simulink model "TorqueVectoringAllocatorTestWrapper"  (R2026b)
settings: Solver=FixedStepDiscrete  StopTime=1.0  FixedStep=TorqueVectoringControlSampleTime
settings Model: DataDictionary=VehicleData.sldd  Creator=Xu Dingyi  LastModifiedBy=29358
settings DebuggingCC: AlgebraicLoopMsg=error

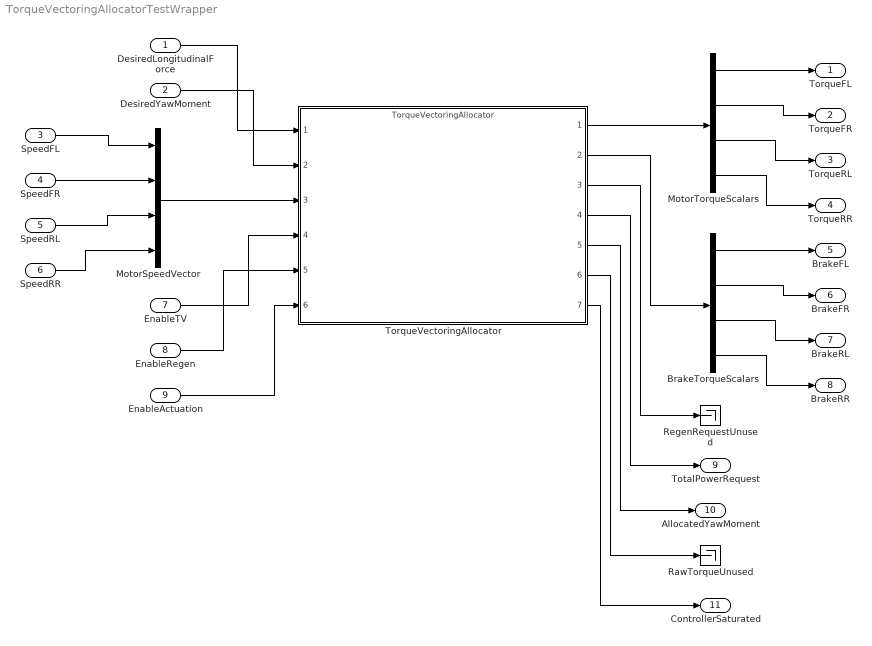
== system TorqueVectoringAllocatorTestWrapper ==
  DesiredLongitudinalForce : Inport  OutDataTypeStr=double  Unit=N
  DesiredYawMoment : Inport  Port=2  OutDataTypeStr=double  Unit=N*m
  SpeedFL : Inport  Port=3  OutDataTypeStr=double  Unit=rad/s
  SpeedFR : Inport  Port=4  OutDataTypeStr=double  Unit=rad/s
  SpeedRL : Inport  Port=5  OutDataTypeStr=double  Unit=rad/s
  SpeedRR : Inport  Port=6  OutDataTypeStr=double  Unit=rad/s
  EnableTV : Inport  Port=7  OutDataTypeStr=boolean
  EnableRegen : Inport  Port=8  OutDataTypeStr=boolean
  EnableActuation : Inport  Port=9  OutDataTypeStr=boolean
  BrakeTorqueScalars : Demux
  MotorSpeedVector : Mux
  MotorTorqueScalars : Demux
  RawTorqueUnused : Terminator
  RegenRequestUnused : Terminator
  TorqueVectoringAllocator : ModelReference  ModelNameDialog=TorqueVectoringAllocator  ModelReferenceVersion=2.0
  TorqueFL : Outport  OutDataTypeStr=double  Unit=N*m
  TorqueFR : Outport  Port=2  OutDataTypeStr=double  Unit=N*m
  TorqueRL : Outport  Port=3  OutDataTypeStr=double  Unit=N*m
  TorqueRR : Outport  Port=4  OutDataTypeStr=double  Unit=N*m
  BrakeFL : Outport  Port=5  OutDataTypeStr=double  Unit=N*m
  BrakeFR : Outport  Port=6  OutDataTypeStr=double  Unit=N*m
  BrakeRL : Outport  Port=7  OutDataTypeStr=double  Unit=N*m
  BrakeRR : Outport  Port=8  OutDataTypeStr=double  Unit=N*m
  TotalPowerRequest : Outport  Port=9  OutDataTypeStr=double  Unit=W
  AllocatedYawMoment : Outport  Port=10  OutDataTypeStr=double  Unit=N*m
  ControllerSaturated : Outport  Port=11  OutDataTypeStr=boolean
  wires:
  SpeedFL/1 -> MotorSpeedVector/1
  MotorSpeedVector/1 -> TorqueVectoringAllocator/3
  SpeedFR/1 -> MotorSpeedVector/2
  TorqueVectoringAllocator/3 -> RegenRequestUnused/1
  DesiredLongitudinalForce/1 -> TorqueVectoringAllocator/1
  SpeedRL/1 -> MotorSpeedVector/3
  EnableTV/1 -> TorqueVectoringAllocator/4
  DesiredYawMoment/1 -> TorqueVectoringAllocator/2
  SpeedRR/1 -> MotorSpeedVector/4
  EnableRegen/1 -> TorqueVectoringAllocator/5
  EnableActuation/1 -> TorqueVectoringAllocator/6
  TorqueVectoringAllocator/1 -> MotorTorqueScalars/1
  TorqueVectoringAllocator/2 -> BrakeTorqueScalars/1
  TorqueVectoringAllocator/4 -> TotalPowerRequest/1
  BrakeTorqueScalars/4 -> BrakeRR/1
  BrakeTorqueScalars/3 -> BrakeRL/1
  TorqueVectoringAllocator/5 -> AllocatedYawMoment/1
  TorqueVectoringAllocator/6 -> RawTorqueUnused/1
  TorqueVectoringAllocator/7 -> ControllerSaturated/1
  MotorTorqueScalars/1 -> TorqueFL/1
  MotorTorqueScalars/2 -> TorqueFR/1
  MotorTorqueScalars/3 -> TorqueRL/1
  MotorTorqueScalars/4 -> TorqueRR/1
  BrakeTorqueScalars/1 -> BrakeFL/1
  BrakeTorqueScalars/2 -> BrakeFR/1
